simulink model "reference_pendulum_setup"  (R2021a)
settings: Solver=FixedStepAuto  StartTime=0.0  StopTime=10  FixedStep=0.01  MaxStep=0.01  RelTol=1e-3
values from neighbouring files (symbols this model uses):
  m = 0.5    [actuated_pendulum_control_analysis.m]
  model_based_control = 1    [demo_noisy_pendulum_data_generation.m]    (also in demo_noisy_pendulum_validation.m = 0)
  s = tf('s')    [actuated_pendulum_control_analysis.m]
undefined symbols (not defined in the file or in its folder): model, policy
libraries: sm_lib x4, nesl_utility x4, simple_link_lib x1
settings Model: Creator=eferr  LastModifiedBy=Enrico
settings SolverCC: AlgebraicLoopSolver=TrustRegion
settings DebuggingCC: SFMachineParentedDataDiag=warning
settings DiagnosticsConfigSet: SimMechanicsUnconnectedFramePorts=none
settings ExplorerConfigSet: InternalSimMechanicsExplorerSettings="<ExplorerConfiguration><canonicalview>planar_xy</canonicalview><AnimationSetting><BasePlaybackSpeed>1.0</BasePlaybackSpeed><PlaybackSpeedFactor>1.0</PlaybackSpeedFactor></AnimationSetting><TilePanel><TileInfo><Tiles Columns=\"1\" Count=\"1\" Rows=\"1\"><Column Weight=\"1\"/><Row Weight=\"1\"/><Tile Height=\"1\" Width=\"1\" X=\"0\" Y=\"0\"/></Tiles></TileInfo><SceneInfo><SceneViewer><BGColor><R>0.60000002384185791</R><G>0.60000002384185791</G><B>0.60000002384185791</B></BGColor><Camera><DoPerspective>off</DoPerspective><Position><X>0.0373521475475569881</X><Y>0.0122054964669870702</Y><Z>1.00000000077561957</Z></Position><Center><X>0.0373521475475569881</X><Y>0.0122054964669870702</Y><Z>7.75619568571528362e-10</Z></Center><Up><X>0</X><Y>1</Y><Z>0</Z></Up><ViewLimDist>1</ViewLimDist><YLim>0.232927452842455418</YLim><XLim>0.430764536165787693</XLim></Camera></SceneViewer></SceneInfo></TilePanel><MechEditorPanel><Cameras/><GfxPanelCameraMap/><VideoCreator><PlaybackSpeedRatio>1.0</PlaybackSpeedRatio><FrameRate>30</FrameRate><VideoFormat>Motion JPEG AVI</VideoFormat><FrameSize>auto</FrameSize></VideoCreator></MechEditorPanel></ExplorerConfiguration>"

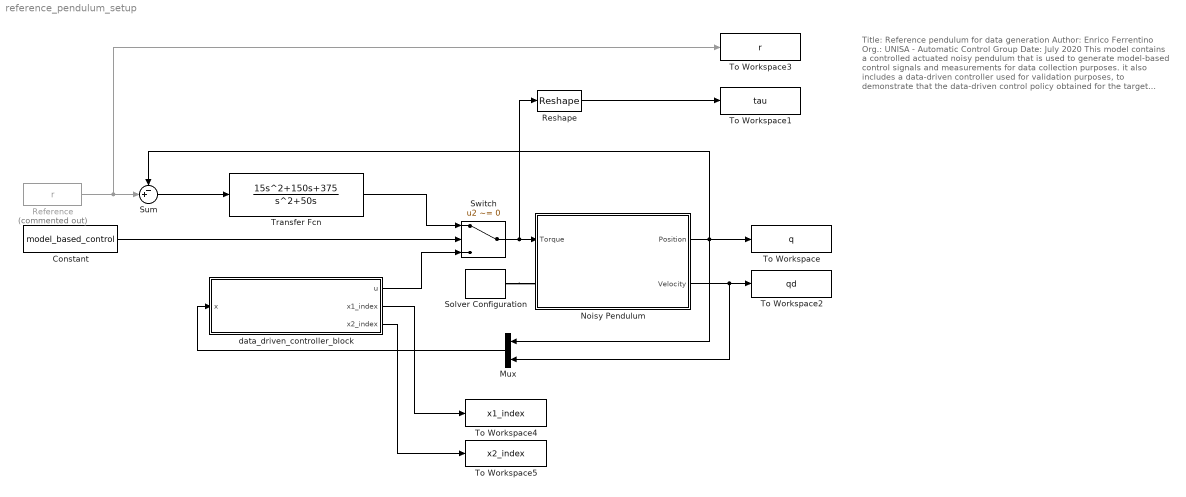
== system reference_pendulum_setup ==
  note: Title: 	Reference pendulum for data generation
      | Author:  	Enrico Ferrentino
      | Org.:     	UNISA - Automatic Control Group
      | Date:     	July 2020
      |
      | This model contains a controlled actuated noisy pendulum that is used
      | to generate model-based control signals and measurements for data
      | collection purposes. it also includes a data-driven controller used for
      | validation purposes, to demonstrate that the data-driven control policy
      | obtained for the target system does not work on the reference system.,
  Constant : Constant  Value=model_based_control
  Mux : Mux  Inputs=2
  Noisy Pendulum : Subsystem  mask{seed=ceil(rand*1000), sigma2=20, sampleTime=0.01}
      mask prompts: sigma2 "Variance"; sampleTime "Simulation step (s)"
  Reference : FromWorkspace  Commented=on  VariableName=r  OutputAfterFinalValue=Holding final value
  Reshape : Reshape  OutputDimensionality=Customize  OutputDimensions=[1]
  Solver Configuration : nesl_utility/Solver Configuration  PhysicalDomain=network_engine_domain  SubClassName=solver  LeftPortType=input  RightPortType=generic  Tones=[]  Harmonics=[]  SimulateNoise=off  Profile=off  UseLocalSampling=off  EnableSwitchedLinearOptims=on  FrequencyDomain=off  UseCCode=off  RelTol=0.001  AbsTol=1e-06  MinStep=1e-09  ToWorkspace=off  RevertToSquareIcSolve=off  NumHomotopyIterations=100  PhasorMode=off  PhasorModeNumHarmonics=1  DoDC=off  ResidualTolerance=1e-09  UseLocalSolver=off  LocalSolverChoice=NE_BACKWARD_EULER_ADVANCER  LocalSolverSampleTime=0.001  DoFixedCost=off  MaxNonlinIter=3  MaxModeIter=2  ComputeImpulses=off  ImpulseIterations=2  LinearAlgebra=auto  EquationFormulation=NE_TIME_EF  DelaysMemoryBudget=1024  AutomaticFiltering=on  FilteringTimeConstant=0.001  PartitionStorageMethod=AS_NEEDED  PartitionMemoryBudget=1024  PartitionMethod=ROBUST
      settings: SourceProductBaseCode=PW,SS
  Sum : Sum  Inputs=-+|
  Switch : Switch  Criteria=u2 ~= 0  Threshold=1
  To Workspace : ToWorkspace  VariableName=q  SaveFormat=Timeseries  SampleTime=-1
  To Workspace1 : ToWorkspace  VariableName=tau  SaveFormat=Timeseries  SampleTime=-1
  To Workspace2 : ToWorkspace  VariableName=qd  SaveFormat=Timeseries  SampleTime=-1
  To Workspace3 : ToWorkspace  VariableName=r  SaveFormat=Timeseries  SampleTime=-1
  To Workspace4 : ToWorkspace  VariableName=x1_index  SaveFormat=Timeseries  SampleTime=-1
  To Workspace5 : ToWorkspace  VariableName=x2_index  SaveFormat=Timeseries  SampleTime=-1
  Transfer Fcn : TransferFcn  Numerator=[15 150 375]  Denominator=[1 50 0]
  data_driven_controller_block : MATLAB Function  TreatAsAtomicUnit=on
  wires:
  Noisy Pendulum/1(Position) -> Mux/1, Sum/1, To Workspace/1
  Transfer Fcn/1 -> Switch/1
  Sum/1 -> Transfer Fcn/1
  Noisy Pendulum/2(Velocity) -> Mux/2, To Workspace2/1
  Reference/1 -> Sum/2, To Workspace3/1
  Reshape/1 -> To Workspace1/1
  Switch/1 -> Reshape/1, Noisy Pendulum/1(Torque)
  data_driven_controller_block/1(u) -> Switch/3
  Constant/1 -> Switch/2
  data_driven_controller_block/2(x1_index) -> To Workspace4/1
  data_driven_controller_block/3(x2_index) -> To Workspace5/1
  Mux/1 -> data_driven_controller_block/1(x)
  connections:
  Solver Configuration/RConn1 -- Noisy Pendulum/LConn1

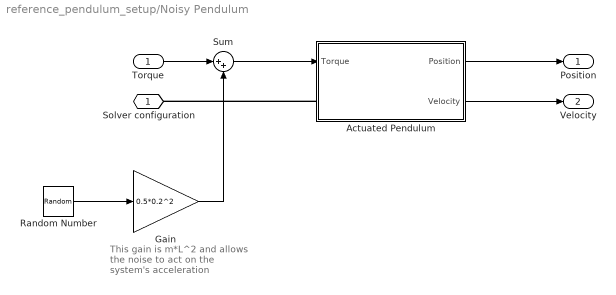
== system reference_pendulum_setup/Noisy Pendulum ==
  note: This gain is m*L^2 and allows the noise to act on the system's acceleration
  Torque : Inport
  Actuated Pendulum : Subsystem
  Gain : Gain  Gain=0.5*0.2^2
  Random Number : RandomNumber  Variance=sigma2  Seed=seed  SampleTime=sampleTime
  Sum : Sum  Inputs=|++
  Solver configuration : PMIOPort  Side=Left
  Position : Outport
  Velocity : Outport  Port=2
  wires:
  Gain/1 -> Sum/2
  Random Number/1 -> Gain/1
  Actuated Pendulum/1(Position) -> Position/1
  Torque/1 -> Sum/1
  Sum/1 -> Actuated Pendulum/1(Torque)
  Actuated Pendulum/2(Velocity) -> Velocity/1
  connections:
  Actuated Pendulum/LConn1 -- Solver configuration/RConn1

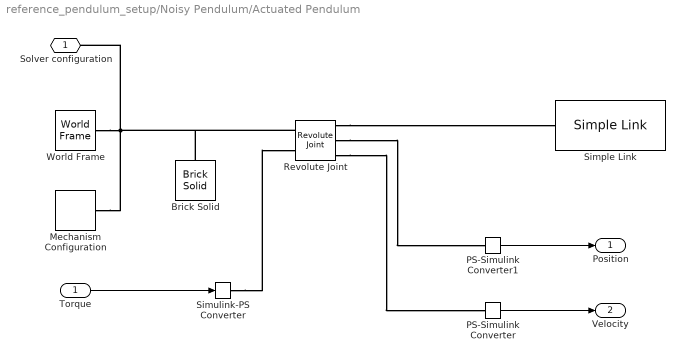
== system reference_pendulum_setup/Noisy Pendulum/Actuated Pendulum ==
  Torque : Inport
  Brick Solid : sm_lib/Body Elements/Brick Solid  GraphicAmbientColor=[0.15 0.15 0.15 1.0]  BasedOnType=Density  BrickDimensions=[4 4 4]  BrickDimensionUnits=cm  CenterOfMass=[0 0 0]  CenterOfMassUnits=m  GraphicDiffuseColor=[0.80 0.45 0]  Density=1000  DensityUnits=kg/m^3  DoExposeReferenceFrame=on  GraphicEmissiveColor=[0.0 0.0 0.0 1.0]  ExportEntireGeometry=off  SerializedFrames=<Frames/>  MarkerShape=Sphere  MarkerSize=10  GraphicType=FromGeometry  InertiaType=CalculateFromGeometry  Mass=1  MassUnits=kg  MomentsOfInertia=[1 1 1]  MomentsOfInertiaUnits=kg*m^2  GraphicOpacity=1.0  ProductsOfInertia=[0 0 0]  ProductsOfInertiaUnits=kg*m^2  GraphicShininess=75  GraphicSpecularColor=[0.5 0.5 0.5 1.0]  GraphicVisPropType=SimpleVisualProperties
  Mechanism Configuration : sm_lib/Utilities/Mechanism Configuration  UniformGravity=Constant  GravityVector=[0 -9.80665 0]  GravityVectorUnits=m/s^2  GravityUnits=m/s^2  LinearizationDelta=0.001  JointModeTransitionNonlinearIterations=2
  PS-Simulink Converter : nesl_utility/PS-Simulink Converter  PhysicalDomain=network_engine_domain  SubClassName=ps_output  LeftPortType=input  RightPortType=output  PseudoPeriodic=off  Frequencies=[]  Unit=inherit  AffineConversion=off
      settings: SourceProductBaseCode=PW,SS
  PS-Simulink Converter1 : nesl_utility/PS-Simulink Converter  PhysicalDomain=network_engine_domain  SubClassName=ps_output  LeftPortType=input  RightPortType=output  PseudoPeriodic=off  Frequencies=[]  Unit=inherit  AffineConversion=off
      settings: SourceProductBaseCode=PW,SS
  Revolute Joint : sm_lib/Joints/Revolute Joint  JointMode=Normal  SenseConstraintForce=off  SenseConstraintForceX=off  SenseConstraintForceY=off  SenseConstraintForceZ=off  SenseConstraintTorque=off  SenseConstraintTorqueX=off  SenseConstraintTorqueY=off  SenseConstraintTorqueZ=off  SenseTotalForce=off  SenseTotalForceX=off  SenseTotalForceY=off  SenseTotalForceZ=off  SenseTotalTorque=off  SenseTotalTorqueX=off  SenseTotalTorqueY=off  SenseTotalTorqueZ=off  CompositeWrenchDir=FollowerOnBase  CompositeWrenchFrame=BaseFrame  EquilibriumPosition=0  EquilibriumPositionUnits=deg  SpringStiffness=0  SpringStiffnessUnits=N*m/deg  DampingCoefficient=8e-5  DampingCoefficientUnits=N*m/(deg/s)  TorqueActuationMode=InputTorque  MotionActuationMode=ComputedMotion  SensePosition=on  SenseVelocity=on  SenseAcceleration=off  SenseTorqueForce=off  SenseLowerLimitTorqueForce=off  SenseUpperLimitTorqueForce=off  LowerLimitSpecify=off  LowerLimitBound=-90  LowerLimitBoundUnits=deg  LowerLimitStiffness=1e4  LowerLimitStiffnessUnits=N*m/deg  LowerLimitDamping=10  LowerLimitDampingUnits=N*m/(deg/s)  LowerLimitTransitionRegionWidth=0.1  LowerLimitTransitionRegionWidthUnits=deg  UpperLimitSpecify=off  UpperLimitBound=90  UpperLimitBoundUnits=deg  UpperLimitStiffness=1e4  UpperLimitStiffnessUnits=N*m/deg  UpperLimitDamping=10  UpperLimitDampingUnits=N*m/(deg/s)  UpperLimitTransitionRegionWidth=0.1  UpperLimitTransitionRegionWidthUnits=deg  PositionTargetSpecify=on  PositionTargetPriority=High  PositionTargetValue=-90  PositionTargetValueUnits=deg  VelocityTargetSpecify=off  VelocityTargetPriority=High  VelocityTargetValue=0  VelocityTargetValueUnits=deg/s
  Simple Link : simple_link_lib/Simple Link  L=20  W=1  H=1  m=0.5  rgb=[0.25 0.40 0.70]
      link override Brick Solid: BasedOnType=Mass  Density=0
  Simulink-PS Converter : nesl_utility/Simulink-PS Converter  PhysicalDomain=network_engine_domain  SubClassName=ps_input  LeftPortType=input  RightPortType=output  PseudoPeriodic=off  Frequencies=[]  NoiseDistribution=none  NoiseParameters=[]  Unit=1  AffineConversion=off  FilteringAndDerivatives=provide  SimscapeFilterOrder=1  InputFilterTimeConstant=0.001  UdotUserProvided=0
      settings: SourceProductBaseCode=PW,SS
  World Frame : sm_lib/Frames and Transforms/World Frame
  Solver configuration : PMIOPort  Side=Left
  Position : Outport
  Velocity : Outport  Port=2
  wires:
  PS-Simulink Converter/1 -> Velocity/1
  Torque/1 -> Simulink-PS Converter/1
  PS-Simulink Converter1/1 -> Position/1
  connections:
  Revolute Joint/RConn3 -- PS-Simulink Converter/LConn1
  Revolute Joint/RConn1 -- Simple Link/LConn1
  Revolute Joint/RConn2 -- PS-Simulink Converter1/LConn1
  Simulink-PS Converter/RConn1 -- Revolute Joint/LConn2
  Mechanism Configuration/RConn1 -- Revolute Joint/LConn1 -- Brick Solid/RConn1 -- Solver configuration/RConn1 -- World Frame/RConn1

== matlab function reference_pendulum_setup/data_driven_controller_block ==
  data: x input; u output; model parameter; policy parameter; x1_index output; x2_index output
function [u, x1_index, x2_index] = data_driven_controller(x, model, policy)

    [min_value, x1_index] = min(abs(model.x1_codebook - x(1)));
    [min_value, x2_index] = min(abs(model.x2_codebook - x(2)));

    [PuM, u_index] = max(policy(1, x1_index, x2_index).Pu);

    u = model.u_codebook(u_index) * model.tau_ref_max;
    
end
